simulink model "MITvd3_9"  (Simulink 7.3)
settings: Solver=ode5  StartTime=0.0  StopTime=100  FixedStep=0.01  RelTol=1e-3
StopFcn:
  | subplot(211);
  | plot(Data.time,Data.signals(1).values(:,1),'r',Data.time,Data.signals(1).values(:,2),'b')
  | subplot(212);
  | plot(Data.time,Data.signals(2).values(:,1),'b')
undefined symbols (not defined in the file or in its folder): b
settings Model: Creator=Minh-Map-Vu  LastModifiedBy=nthuy
settings DataIOCC: SignalLoggingName=sigsOut
settings DebuggingCC: SaveWithParameterizedLinksMsg=none  SignalResolutionControl=TryResolveAllWithWarning  SolverPrmCheckMsg=none  MultiTaskDSMMsg=warning  MultiTaskCondExecSysMsg=none  StrictBusMsg=None
settings HardwareCC: TargetEndianess=LittleEndian  TargetHWDeviceType=MATLAB Host  ProdEqTarget=off
settings RTWCC: IncludeERTFirstTime=on

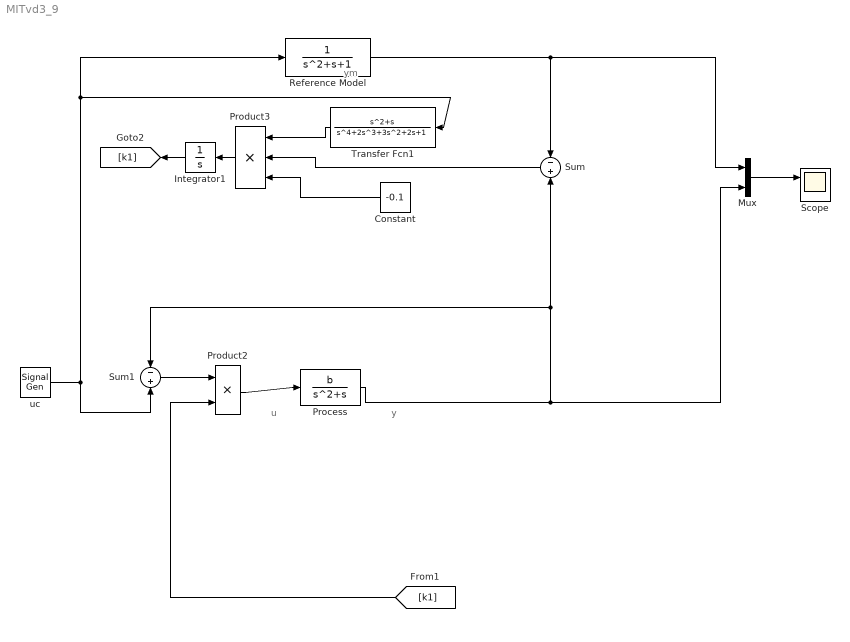
== system MITvd3_9 ==
  note: ym
  note: u
  note: y
  Constant : Constant  Value=-0.1  OutDataType=fixdt(1, 16)  OutScaling=2^0
  Integrator1 : Integrator
  Mux : Mux  Inputs=2
  Process : TransferFcn  Numerator=b  Denominator=[1 1 0]
  Product2 : Product  SaturateOnIntegerOverflow=on  OutDataTypeStr=Inherit: Same as first input
  Product3 : Product  Inputs=3  SaturateOnIntegerOverflow=on  OutDataTypeStr=Inherit: Same as first input
  Reference Model : TransferFcn  Denominator=[1 1 1]
  Scope : Scope  NumInputPorts=2
      settings: TimeRange=100  YMin=-1.2~-5  YMax=1.2~5  SaveName=Data
  Sum : Sum  Inputs=-+  SaturateOnIntegerOverflow=on
  Sum1 : Sum  Inputs=-+  SaturateOnIntegerOverflow=on
  Transfer Fcn1 : TransferFcn  Numerator=[1 1 0]  Denominator=[1 2 3 2 1]
  uc : SignalGenerator  WaveForm=square  Frequency=1/20
  wires:
  uc/1 -> Reference Model/1, Transfer Fcn1/1, Sum1/2
  Reference Model/1 -> Sum/1, Mux/1
  Process/1 -> Mux/2, Sum/2, Sum1/1
  Mux/1 -> Scope/1
  Product3/1 -> Integrator1/1
  Transfer Fcn1/1 -> Product3/1
  Constant/1 -> Product3/3
  Integrator1/1 -> [k1]
  Sum/1 -> Product3/2
  [k1] -> Product2/2
  Sum1/1 -> Product2/1
  Product2/1 -> Process/1
